simulink model "BrakeSimProto"  (R2023a)
settings: Solver=ode4  StartTime=0.0  StopTime=10.0  FixedStep=0.000000095238  RelTol=1e-3
values from neighbouring files (symbols this model uses):
  Control = 0    [SimProgram.m]    (also in bike_absdata.m = 1)
  g = 32.18    [bike_absdata.m]
  m = 50    [bike_absdata.m]
  mu = [0 .4 .8 .97 1.0 .98 .96 .94 .92 .9 .88 .855 .83 .81 .79 .77 .75 .73 .72 .71 .7]    [bike_absdata.m]
  r = 0.90    (= 0.9)    [bike_absdata.m]
  slip = (0:.05:1.0)    [bike_absdata.m]
settings Model: Creator=ecc5  LastModifiedBy=ecc5
settings OptimizationCC: DefaultParameterBehavior=Inlined  EnhancedBackFolding=on  PassReuseOutputArgsAs=Individual arguments  ZeroExternalMemoryAtStartup=off  ZeroInternalMemoryAtStartup=off  OptimizeBlockOrder=speed  DifferentSizesBufferReuse=on  OptimizationCustomize=off  EfficientTunableParamExpr=on
settings DebuggingCC: ParameterTunabilityLossMsg=error
settings SFSimCC: MATLABDynamicMemAlloc=off
settings RTWCC: Description=Embedded Coder  SystemTargetFile=ert.tlc  TemplateMakefile=ert_default_tmf
settings CodeAppCC: ForceParamTrailComments=on  IgnoreCustomStorageClasses=off  OperatorAnnotations=on  SimulinkDataObjDesc=on  SFDataObjDesc=on  InsertBlockDesc=on
settings ERTTargetCC: TargetLangStandard=C99 (ISO)  GenerateSampleERTMain=on  InlinedParameterPlacement=NonHierarchical  ERTCustomFileTemplate=example_file_process.tlc

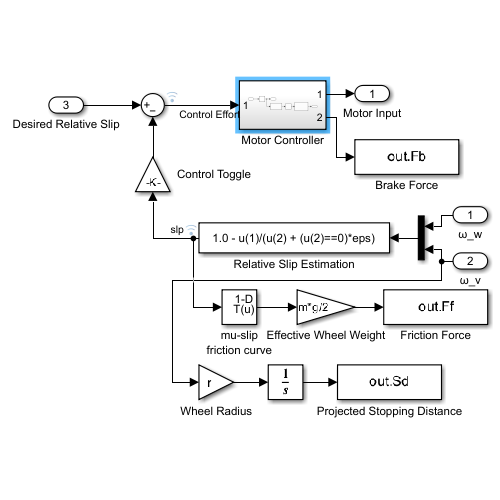
[thumbnail: Simulink's stored preview of the top-level diagram]
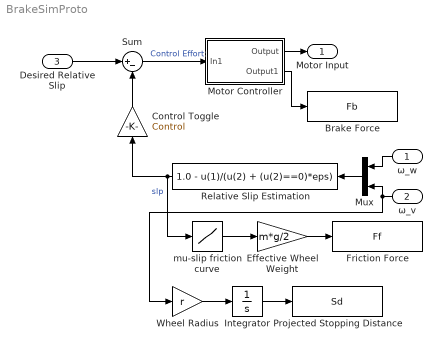
== system BrakeSimProto ==
  ω_w : Inport
  ω_v : Inport  Port=2
  Desired Relative Slip : Inport  Port=3
  Brake Force : ToWorkspace  VariableName=Fb  SaveFormat=Timeseries  SampleTime=-1
  Control Toggle : Gain  Gain=Control
  Effective Wheel Weight : Gain  Gain=m*g/2
  Friction Force : ToWorkspace  VariableName=Ff  SaveFormat=Timeseries  SampleTime=-1
  Integrator : Integrator
  Motor Controller : Subsystem
  Mux : Mux  Inputs=2
  Projected Stopping Distance : ToWorkspace  VariableName=Sd  SaveFormat=Timeseries  SampleTime=-1
  Relative Slip Estimation : Fcn  Expr=1.0 - u(1)/(u(2) + (u(2)==0)*eps)
  Sum : Sum  Inputs=|+-
  Wheel Radius : Gain  Gain=r
  mu-slip friction curve : Lookup_n-D  NumberOfTableDimensions=1  BreakpointsForDimension1=slip  Table=mu  SaturateOnIntegerOverflow=on
  Motor Input : Outport
  wires:
  Desired Relative Slip/1 -> Sum/1
  Control Toggle/1 -> Sum/2
  Mux/1 -> Relative Slip Estimation/1
  ω_w/1 -> Mux/1
  ω_v/1 -> Wheel Radius/1, Mux/2
  Relative Slip Estimation/1 -> mu-slip friction curve/1, Control Toggle/1  "slp"
  mu-slip friction curve/1 -> Effective Wheel Weight/1
  Effective Wheel Weight/1 -> Friction Force/1
  Wheel Radius/1 -> Integrator/1
  Integrator/1 -> Projected Stopping Distance/1
  Motor Controller/2(Output1) -> Brake Force/1
  Sum/1 -> Motor Controller/1(In1)  "Control Effort"
  Motor Controller/1(Output) -> Motor Input/1

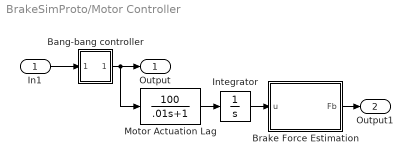
== system BrakeSimProto/Motor Controller ==
  In1 : Inport
  Bang-bang controller : Subsystem  mask(Sign){}
      mask help: y = sign(x)
      mask Help: Sign Function:\n\t\t\ty = 1 if x > 0\n\t\t\ty = 0 if x = 0\n\t\t\ty = -1 if x < 0
      mask Display: plot(-50,-50,50,50,[-50,50],[0,0],[0,0],[-50,50],[-40,0],[-30,-30],[0,40],[30,30])
  Brake Force Estimation : MATLAB Function  TreatAsAtomicUnit=on
  Integrator : Integrator
  Motor Actuation Lag : TransferFcn  Numerator=[100]  Denominator=[.01 1]
  Output : Outport
  Output1 : Outport  Port=2
  wires:
  In1/1 -> Bang-bang controller/1(in_1)
  Integrator/1 -> Brake Force Estimation/1(u)
  Brake Force Estimation/1(Fb) -> Output1/1
  Motor Actuation Lag/1 -> Integrator/1
  Bang-bang controller/1(out_1) -> Motor Actuation Lag/1, Output/1

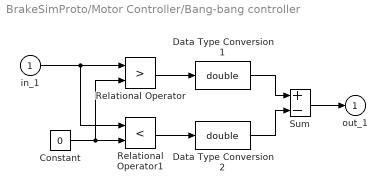
== system BrakeSimProto/Motor Controller/Bang-bang controller ==
  in_1 : Inport
  Constant : Constant  Value=0
  Data Type Conversion1 : DataTypeConversion  OutDataTypeStr=double
  Data Type Conversion2 : DataTypeConversion  OutDataTypeStr=double
  Relational Operator : RelationalOperator  Operator=>  OutDataTypeStr=boolean
  Relational Operator1 : RelationalOperator  Operator=<  OutDataTypeStr=boolean
  Sum : Sum  Inputs=+-  InputSameDT=on  SaturateOnIntegerOverflow=on  OutDataTypeStr=Inherit: Same as first input
  out_1 : Outport  InitialOutput=0  VectorParamsAs1DForOutWhenUnconnected=off
  wires:
  Data Type Conversion2/1 -> Sum/2
  Data Type Conversion1/1 -> Sum/1
  Sum/1 -> out_1/1
  Relational Operator/1 -> Data Type Conversion1/1
  Relational Operator1/1 -> Data Type Conversion2/1
  Constant/1 -> Relational Operator/2, Relational Operator1/2
  in_1/1 -> Relational Operator1/1, Relational Operator/1

== matlab function BrakeSimProto/Motor Controller/Brake Force Estimation ==
  data: u input; Fb output
function Fb = fcn(u)

k1 = 0.7;
k2 = 0.23;

Fb = k1*k2*u - 0.6;
